simulink model "ForceBounding"  (Simulink 8.6)
settings: Solver=VariableStepAuto  StartTime=0.0  StopTime=50  RelTol=1e-3
values from neighbouring files (symbols this model uses):
  bDevice = block.DialogPrm(1).Data    [Controller.m]    (also in Controller1.m; LessConservative.m; MoreConservative.m; Parameters.m = 0.1)
  mDevice = 0.1    [Parameters.m]
  p0 = block.DialogPrm(4).Data    [Controller.m]    (also in Controller1.m; Initiation.m = 0.12; Parameters.m = 1; VirtualEnvironment.m = block.DialogPrm(8).Data)
  v0 = block.DialogPrm(6).Data    [HapticDevice.m]    (also in HumanOperator.m; Initiation.m = 0; Parameters.m = 0; VirtualEnvironment4.m = block.DialogPrm(8).Data)
settings Model: Creator=TOSHIBA  LastModifiedBy=TOSHIBA
settings DataIOCC: SaveFormat=Dataset  SignalLoggingSaveFormat=Dataset
settings OptimizationCC: ExpressionDepthLimit=128
settings DebuggingCC: UnderspecifiedInitializationDetection=Simplified  MergeDetectMultiDrivingBlocksExec=error  SolverPrmCheckMsg=none  FcnCallInpInsideContextMsg=EnableAllAsError  StateNameClashWarn=none
settings HardwareCC: ProdBitPerPointer=64  ProdLargestAtomicFloat=Float  ProdIntDivRoundTo=Zero  ProdEndianess=LittleEndian  ProdWordSize=64  ProdHWDeviceType=Intel->x86-64 (Windows64)
settings GRTTargetCC: GeneratePreprocessorConditionals=Use local settings  CombineOutputUpdateFcns=on  GRTInterface=off
settings ConfigComp: CovModelRefEnable=off

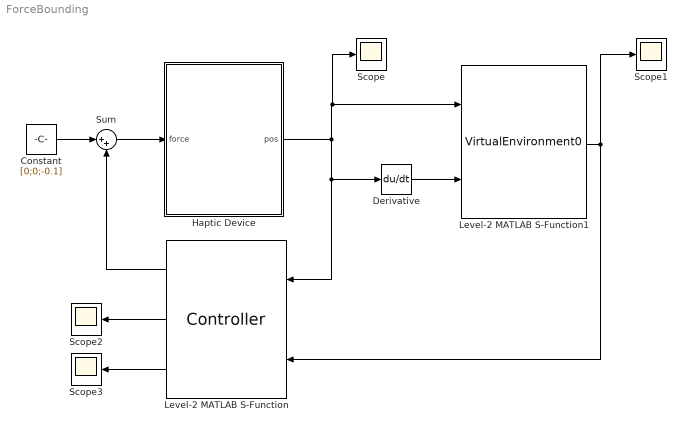
== system ForceBounding ==
  Constant : Constant  Value=[0;0;-0.1]
  Derivative : Derivative
  Haptic Device : Subsystem
  Level-2 MATLAB S-Function : M-S-Function  FunctionName=Controller  Parameters=bDevice, dof, tsampling, p0
  Level-2 MATLAB S-Function1 : M-S-Function  FunctionName=VirtualEnvironment0  Parameters=kBall, bBall, nBall, cBall, rBall, dof, tsampling
  Scope{,1..3} (4 alike) : Scope
  Sum : Sum  Inputs=|++
  wires:
  Derivative/1 -> Level-2 MATLAB S-Function1/2
  Haptic Device/1(pos) -> Scope/1, Level-2 MATLAB S-Function1/1, Level-2 MATLAB S-Function/1, Derivative/1
  Level-2 MATLAB S-Function1/1 -> Level-2 MATLAB S-Function/2, Scope1/1
  Sum/1 -> Haptic Device/1(force)
  Constant/1 -> Sum/1
  Level-2 MATLAB S-Function/2 -> Scope2/1
  Level-2 MATLAB S-Function/3 -> Scope3/1
  Level-2 MATLAB S-Function/1 -> Sum/2

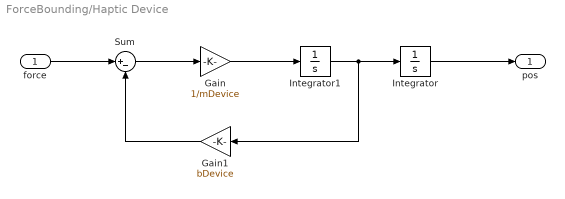
== system ForceBounding/Haptic Device ==
  force : Inport
  Gain : Gain  Gain=1/mDevice
  Gain1 : Gain  Gain=bDevice
  Integrator : Integrator  InitialCondition=p0
  Integrator1 : Integrator  InitialCondition=v0
  Sum : Sum  Inputs=|+-
  pos : Outport
  wires:
  Gain1/1 -> Sum/2
  force/1 -> Sum/1
  Integrator/1 -> pos/1
  Sum/1 -> Gain/1
  Integrator1/1 -> Gain1/1, Integrator/1
  Gain/1 -> Integrator1/1
